simulink model "mass_spring_damper"  (R2019a)
settings: Solver=VariableStepAuto  StartTime=0.0  StopTime=200.0  RelTol=1e-3
model workspace (MAT data in the model file):
  F = 1
  c = 10
  d = 1
  m = 10
settings Model: Creator=evgheniivolodscoi  LastModifiedBy=evgheniivolodscoi

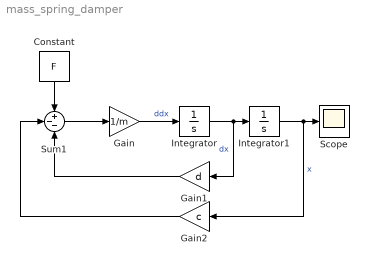
== system mass_spring_damper ==
  Constant : Constant  Value=F
  Gain : Gain  Gain=1/m
  Gain1 : Gain  Gain=d
  Gain2 : Gain  Gain=c
  Integrator : Integrator
  Integrator1 : Integrator  InitialCondition=2
  Scope : Scope
  Sum1 : Sum  Inputs=+--
  wires:
  Sum1/1 -> Gain/1
  Constant/1 -> Sum1/1
  Gain/1 -> Integrator/1  "ddx"
  Integrator/1 -> Gain1/1, Integrator1/1  "dx"
  Integrator1/1 -> Gain2/1, Scope/1  "x"
  Gain1/1 -> Sum1/3
  Gain2/1 -> Sum1/2
